simulink subsystem "PvtSubSys_AHBC"  (R2020b)
settings: Solver=VariableStepAuto  StartTime=0.0  StopTime=10.0  RelTol=1e-3
undefined symbols (not defined in the file): P_AHBC_ABS_ENABLE, P_AHBC_DRIVE_DIRECTION_ENABLE, P_AHBC_ESP_ENABLE, P_AHBC_FOG_ENABLE, P_AHBC_FOG_TIME, P_AHBC_HIGHBEAM_ACTIVE_GRACE, P_AHBC_LAT_ACC_ENTER, P_AHBC_LAT_ACC_EXIT, P_AHBC_MAX_ONCOMING_DISTANCE_COUPLE2, P_AHBC_MAX_ONCOMING_DISTANCE_ONE2, P_AHBC_MAX_TAILLIGHT_DISTANCE_COUPLE2, P_AHBC_MAX_TAILLIGHT_DISTANCE_ONE2, P_AHBC_SPEED_SWITCH_HIGH_BEAM_OFF2, P_AHBC_SPEED_SWITCH_HIGH_BEAM_ON2, P_AHBC_TrafficStyle, P_AHBC_TURN_LAMP_ENABLE, P_AHBC_WIPER_ENABLE, P_AHBC_WIPER_TIME, P_AHBC_YAW_RATE_ENTER, P_AHBC_YAW_RATE_EXIT
libraries: simulink x57
(part 3 of 4)

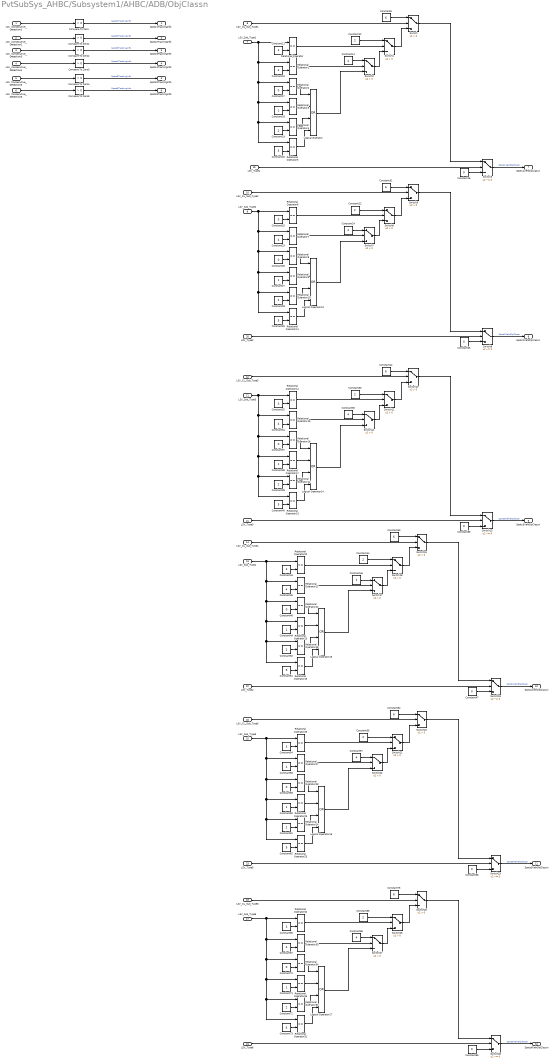
== system PvtSubSys_AHBC/Subsystem1/AHBC/ADB/ObjClassn ==
  LSV_Consecutive_Detection1 : Inport
  LSV_Consecutive_Detection2 : Inport  Port=2
  LSV_Consecutive_Detection3 : Inport  Port=3
  LSV_Consecutive_Detection4 : Inport  Port=4
  LSV_Consecutive_Detection5 : Inport  Port=5
  LSV_Consecutive_Detection6 : Inport  Port=6
  LSV_Sub_Type1 : Inport  Port=7
  LSV_CL_Sub_Type1 : Inport  Port=8
  LSV_Sub_Type2 : Inport  Port=9
  LSV_CL_Sub_Type2 : Inport  Port=10
  LSV_Sub_Type3 : Inport  Port=11
  LSV_CL_Sub_Type3 : Inport  Port=12
  LSV_Sub_Type4 : Inport  Port=13
  LSV_CL_Sub_Type4 : Inport  Port=14
  LSV_Sub_Type5 : Inport  Port=15
  LSV_CL_Sub_Type5 : Inport  Port=16
  LSV_Sub_Type6 : Inport  Port=17
  LSV_CL_Sub_Type6 : Inport  Port=18
  LSV_Type1 : Inport  Port=19
  LSV_Type2 : Inport  Port=20
  LSV_Type3 : Inport  Port=21
  LSV_Type4 : Inport  Port=22
  LSV_Type5 : Inport  Port=23
  LSV_Type6 : Inport  Port=24
  Compare To Zero{,1..5} (6 alike) : simulink/Logic and Bit Operations/Compare To Zero  relop=>  OutDataTypeStr=boolean
  Constant{11,15,32,43,54,65} (6 alike) : Constant  Value=3
  Constant{12,19,22,28,33,39,44,50,55,61,66,72} (12 alike) : Constant  Value=2
  Constant{13..14,23..24,34..35,45..46,56..57,67..68} (12 alike) : Constant  Value=4
  Constant{16..17,25..26,36..37,47..48,58..59,69..70} (12 alike) : Constant  Value=0
  Constant{18,27,38,49,60,71} (6 alike) : Constant
  Constant{20,29,40,51,62,73} (6 alike) : Constant  Value=5
  Constant{6,31,42,53,64,75} (6 alike) : Constant  Value=6
  Logical Operator{,13..17} (6 alike) : Logic  Operator=OR  Inputs=4  AllPortsSameDT=off  OutDataTypeStr=boolean
  Relational Operator{,1..35} (36 alike) : RelationalOperator  Operator===  OutDataTypeStr=boolean  RndMeth=Simplest
  Switch{,1..2,5..7,10..12,15..17,20..22,25..27} (18 alike) : Switch  Criteria=u2 > Threshold  OutDataTypeStr=uint8
  Switch{3,8,13,18,23,28} (6 alike) : Switch  Criteria=u2 ~= 0  OutDataTypeStr=uint8
  Spots1TrackingInfo : Outport  OutDataTypeStr=boolean  PortDimensions=1
  Spots2TrackingInfo : Outport  Port=2  OutDataTypeStr=boolean  PortDimensions=1
  Spots3TrackingInfo : Outport  Port=3  OutDataTypeStr=boolean  PortDimensions=1
  Spots4TrackingInfo : Outport  Port=4  OutDataTypeStr=boolean  PortDimensions=1
  Spots5TrackingInfo : Outport  Port=5  OutDataTypeStr=boolean  PortDimensions=1
  Spots6TrackingInfo : Outport  Port=6  OutDataTypeStr=boolean  PortDimensions=1
  Spots1VehObjClassn : Outport  Port=7  OutDataTypeStr=uint8  PortDimensions=1
  Spots2VehObjClassn : Outport  Port=8  OutDataTypeStr=uint8  PortDimensions=1
  Spots3VehObjClassn : Outport  Port=9  OutDataTypeStr=uint8  PortDimensions=1
  Spots4VehObjClassn : Outport  Port=10  OutDataTypeStr=uint8  PortDimensions=1
  Spots5VehObjClassn : Outport  Port=11  OutDataTypeStr=uint8  PortDimensions=1
  Spots6VehObjClassn : Outport  Port=12  OutDataTypeStr=uint8  PortDimensions=1
  wires:
  LSV_Consecutive_Detection4/1 -> Compare To Zero3/1
  Compare To Zero3/1 -> Spots4TrackingInfo/1  "Spots4TrackingInfo"
  Compare To Zero4/1 -> Spots5TrackingInfo/1  "Spots5TrackingInfo"
  LSV_Consecutive_Detection5/1 -> Compare To Zero4/1
  LSV_Consecutive_Detection6/1 -> Compare To Zero5/1
  Compare To Zero5/1 -> Spots6TrackingInfo/1  "Spots6TrackingInfo"
  Compare To Zero2/1 -> Spots3TrackingInfo/1  "Spots3TrackingInfo"
  LSV_Consecutive_Detection3/1 -> Compare To Zero2/1
  LSV_Consecutive_Detection2/1 -> Compare To Zero1/1
  Compare To Zero1/1 -> Spots2TrackingInfo/1  "Spots2TrackingInfo"
  Compare To Zero/1 -> Spots1TrackingInfo/1  "Spots1TrackingInfo"
  LSV_Consecutive_Detection1/1 -> Compare To Zero/1
  Logical Operator17/1 -> Switch27/3
  Logical Operator16/1 -> Switch22/3
  Logical Operator15/1 -> Switch17/3
  Logical Operator14/1 -> Switch12/3
  Logical Operator13/1 -> Switch7/3
  Logical Operator/1 -> Switch2/3
  Constant69/1 -> Switch28/3
  Switch21/1 -> Switch20/3
  Relational Operator29/1 -> Logical Operator16/2
  Relational Operator28/1 -> Logical Operator16/1
  Switch28/1 -> Spots6VehObjClassn/1  "Spots6VehObjClassn"
  Constant31/1 -> Switch5/1
  Relational Operator34/1 -> Logical Operator17/1
  LSV_Type4/1 -> Switch18/2
  Relational Operator30/1 -> Logical Operator17/3
  Constant71/1 -> Relational Operator35/2
  Constant56/1 -> Relational Operator27/2
  Relational Operator24/1 -> Logical Operator16/3
  Constant61/1 -> Relational Operator24/2
  Relational Operator22/1 -> Logical Operator15/1
  Switch22/1 -> Switch21/3
  Constant73/1 -> Relational Operator31/2
  Switch6/1 -> Switch5/3
  Relational Operator9/1 -> Logical Operator13/2
  Constant54/1 -> Relational Operator26/2
  Constant64/1 -> Switch20/1
  Constant24/1 -> Switch7/1
  Constant53/1 -> Switch15/1
  Switch15/1 -> Switch18/1
  Constant45/1 -> Relational Operator21/2
  Switch23/1 -> Spots5VehObjClassn/1  "Spots5VehObjClassn"
  Switch16/1 -> Switch15/3
  Constant47/1 -> Switch18/3
  Constant48/1 -> Relational Operator22/2
  Relational Operator13/1 -> Logical Operator14/4
  LSV_CL_Sub_Type5/1 -> Switch20/2
  Relational Operator12/1 -> Logical Operator14/3
  Relational Operator16/1 -> Logical Operator14/1
  Relational Operator17/1 -> Logical Operator14/2
  Relational Operator4/1 -> Logical Operator/3
  Constant58/1 -> Switch23/3
  Relational Operator18/1 -> Logical Operator15/3
  Constant36/1 -> Switch13/3
  LSV_CL_Sub_Type6/1 -> Switch25/2
  LSV_Type6/1 -> Switch28/2
  Relational Operator23/1 -> Logical Operator15/2
  Constant38/1 -> Relational Operator17/2
  Constant65/1 -> Relational Operator32/2
  Constant70/1 -> Relational Operator34/2
  LSV_Sub_Type2/1 -> Relational Operator6/1, Relational Operator7/1, Relational Operator8/1, Relational Operator9/1, Relational Operator11/1, Relational Operator10/1
  LSV_Type1/1 -> Switch3/2
  Constant62/1 -> Relational Operator25/2
  LSV_Sub_Type6/1 -> Relational Operator32/1, Relational Operator33/1, Relational Operator34/1, Relational Operator35/1, Relational Operator31/1, Relational Operator30/1
  Constant23/1 -> Relational Operator7/2
  Relational Operator27/1 -> Switch22/2
  Constant26/1 -> Relational Operator8/2
  LSV_Type3/1 -> Switch13/2
  Constant6/1 -> Switch/1
  Relational Operator31/1 -> Logical Operator17/4
  Constant50/1 -> Relational Operator18/2
  LSV_CL_Sub_Type2/1 -> Switch5/2
  Constant20/1 -> Relational Operator5/2
  Constant68/1 -> Switch27/1
  LSV_Type5/1 -> Switch23/2
  Relational Operator10/1 -> Logical Operator13/3
  Constant32/1 -> Relational Operator14/2
  Relational Operator21/1 -> Switch17/2
  Switch11/1 -> Switch10/3
  Constant46/1 -> Switch17/1
  Switch27/1 -> Switch26/3
  Constant60/1 -> Relational Operator29/2
  Constant72/1 -> Relational Operator30/2
  Relational Operator8/1 -> Logical Operator13/1
  Constant57/1 -> Switch22/1
  Constant25/1 -> Switch8/3
  Constant16/1 -> Switch3/3
  Switch7/1 -> Switch6/3
  Switch5/1 -> Switch8/1
  Switch18/1 -> Spots4VehObjClassn/1  "Spots4VehObjClassn"
  Switch20/1 -> Switch23/1
  Constant39/1 -> Relational Operator12/2
  Constant33/1 -> Switch11/1
  Constant37/1 -> Relational Operator16/2
  LSV_Sub_Type1/1 -> Relational Operator4/1, Relational Operator5/1, Relational Operator3/1, Relational Operator2/1, Relational Operator1/1, Relational Operator/1
  Constant42/1 -> Switch10/1
  Relational Operator25/1 -> Logical Operator16/4
  Switch13/1 -> Spots3VehObjClassn/1  "Spots3VehObjClassn"
  Constant27/1 -> Relational Operator9/2
  Relational Operator15/1 -> Switch12/2
  Switch17/1 -> Switch16/3
  Constant22/1 -> Switch6/1
  LSV_Sub_Type4/1 -> Relational Operator20/1, Relational Operator21/1, Relational Operator22/1, Relational Operator23/1, Relational Operator19/1, Relational Operator18/1
  Constant15/1 -> Relational Operator6/2
  Switch26/1 -> Switch25/3
  Relational Operator7/1 -> Switch7/2
  Constant28/1 -> Relational Operator10/2
  Constant67/1 -> Relational Operator33/2
  Constant44/1 -> Switch16/1
  Relational Operator11/1 -> Logical Operator13/4
  Constant51/1 -> Relational Operator19/2
  Constant12/1 -> Switch1/1
  Relational Operator5/1 -> Logical Operator/4
  Relational Operator3/1 -> Logical Operator/2
  Constant43/1 -> Relational Operator20/2
  LSV_Type2/1 -> Switch8/2
  Switch10/1 -> Switch13/1
  Constant19/1 -> Relational Operator4/2
  Relational Operator33/1 -> Switch27/2
  Switch3/1 -> Spots1VehObjClassn/1  "Spots1VehObjClassn"
  Relational Operator6/1 -> Switch6/2
  Constant35/1 -> Switch12/1
  Switch12/1 -> Switch11/3
  Relational Operator2/1 -> Logical Operator/1
  Switch8/1 -> Spots2VehObjClassn/1  "Spots2VehObjClassn"
  Relational Operator32/1 -> Switch26/2
  Relational Operator26/1 -> Switch21/2
  Constant18/1 -> Relational Operator3/2
  Relational Operator19/1 -> Logical Operator15/4
  Relational Operator14/1 -> Switch11/2
  Switch1/1 -> Switch/3
  Constant17/1 -> Relational Operator2/2
  Constant40/1 -> Relational Operator13/2
  LSV_Sub_Type3/1 -> Relational Operator12/1, Relational Operator13/1, Relational Operator17/1, Relational Operator16/1, Relational Operator15/1, Relational Operator14/1
  Constant49/1 -> Relational Operator23/2
  Constant14/1 -> Switch2/1
  Switch2/1 -> Switch1/3
  Relational Operator20/1 -> Switch16/2
  LSV_CL_Sub_Type3/1 -> Switch10/2
  Constant55/1 -> Switch21/1
  Constant75/1 -> Switch25/1
  Constant66/1 -> Switch26/1
  Switch/1 -> Switch3/1
  Constant11/1 -> Relational Operator/2
  LSV_CL_Sub_Type1/1 -> Switch/2
  LSV_CL_Sub_Type4/1 -> Switch15/2
  Relational Operator35/1 -> Logical Operator17/2
  Constant13/1 -> Relational Operator1/2
  Constant59/1 -> Relational Operator28/2
  Constant34/1 -> Relational Operator15/2
  Switch25/1 -> Switch28/1
  Relational Operator/1 -> Switch1/2
  Constant29/1 -> Relational Operator11/2
  LSV_Sub_Type5/1 -> Relational Operator24/1, Relational Operator25/1, Relational Operator29/1, Relational Operator28/1, Relational Operator27/1, Relational Operator26/1
  Relational Operator1/1 -> Switch2/2

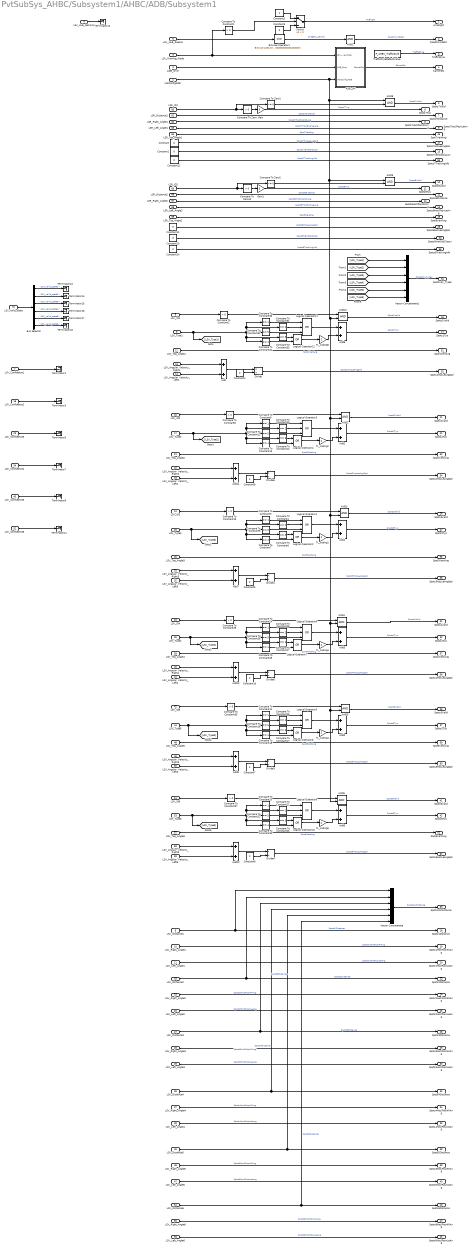
== system PvtSubSys_AHBC/Subsystem1/AHBC/ADB/Subsystem1 ==
  VehConfigADB : Inport
  ADB_error : Inport  Port=2
  LSV_Running_Mode : Inport  Port=3
  LSV_HLB_Decision : Inport  Port=4
  LSV_HLB_Reason : Inport  Port=5
  LSV_ID1 : Inport  Port=6
  LSV_Confidence1 : Inport  Port=7
  LSV_Type1 : Inport  Port=8
  LSV_Distance1 : Inport  Port=9  OutDataTypeStr=uint16
  LSV_Right_Angle1 : Inport  Port=10
  LSV_Left_Angle1 : Inport  Port=11
  LSV_Top_Angle1 : Inport  Port=12
  LSV_Angular_Velocity_Right1 : Inport  Port=13
  LSV_Angular_Velocity_Left1 : Inport  Port=14
  LSV_ID2 : Inport  Port=15
  LSV_Confidence2 : Inport  Port=16
  LSV_Type2 : Inport  Port=17
  LSV_Distance2 : Inport  Port=18  OutDataTypeStr=uint16
  LSV_Right_Angle2 : Inport  Port=19
  LSV_Left_Angle2 : Inport  Port=20
  LSV_Top_Angle2 : Inport  Port=21
  LSV_Angular_Velocity_Right2 : Inport  Port=22
  LSV_Angular_Velocity_Left2 : Inport  Port=23
  LSV_ID3 : Inport  Port=24
  LSV_Confidence3 : Inport  Port=25
  LSV_Type3 : Inport  Port=26
  LSV_Distance3 : Inport  Port=27  OutDataTypeStr=uint16
  LSV_Right_Angle3 : Inport  Port=28
  LSV_Left_Angle3 : Inport  Port=29
  LSV_Top_Angle3 : Inport  Port=30
  LSV_Angular_Velocity_Right3 : Inport  Port=31
  LSV_Angular_Velocity_Left3 : Inport  Port=32
  LSV_ID4 : Inport  Port=33
  LSV_Confidence4 : Inport  Port=34
  LSV_Type4 : Inport  Port=35
  LSV_Distance4 : Inport  Port=36  OutDataTypeStr=uint16
  LSV_Right_Angle4 : Inport  Port=37
  LSV_Left_Angle4 : Inport  Port=38
  LSV_Top_Angle4 : Inport  Port=39
  LSV_Angular_Velocity_Right4 : Inport  Port=40
  LSV_Angular_Velocity_Left4 : Inport  Port=41
  LSV_ID5 : Inport  Port=42
  LSV_Confidence5 : Inport  Port=43
  LSV_Type5 : Inport  Port=44
  LSV_Distance5 : Inport  Port=45  OutDataTypeStr=uint16
  LSV_Right_Angle5 : Inport  Port=46
  LSV_Left_Angle5 : Inport  Port=47
  LSV_Top_Angle5 : Inport  Port=48
  LSV_Angular_Velocity_Right5 : Inport  Port=49
  LSV_Angular_Velocity_Left5 : Inport  Port=50
  LSV_ID6 : Inport  Port=51
  LSV_Confidence6 : Inport  Port=52
  LSV_Type6 : Inport  Port=53
  LSV_Distance6 : Inport  Port=54  OutDataTypeStr=uint16
  LSV_Right_Angle6 : Inport  Port=55
  LSV_Left_Angle6 : Inport  Port=56
  LSV_Top_Angle6 : Inport  Port=57
  LSV_Angular_Velocity_Right6 : Inport  Port=58
  LSV_Angular_Velocity_Left6 : Inport  Port=59
  LSR_ID1 : Inport  Port=60
  LSR_Distance1 : Inport  Port=61  OutDataTypeStr=uint16
  LSR_Right_Angle1 : Inport  Port=62
  LSR_Left_Angle1 : Inport  Port=63
  LSR_Top_Angle1 : Inport  Port=64
  LSR_ID2 : Inport  Port=65
  LSR_Distance2 : Inport  Port=66  OutDataTypeStr=uint16
  LSR_Right_Angle2 : Inport  Port=67
  LSR_Left_Angle2 : Inport  Port=68
  LSR_Top_Angle2 : Inport  Port=69
  LSV_valid_state : Inport  Port=70
  ADB_SM : Stateflow chart  TreatAsAtomicUnit=on
  AND1 : Logic  Inputs=1  AllPortsSameDT=off  OutDataTypeStr=boolean
  AND{2..6,8..10} (8 alike) : Logic  AllPortsSameDT=off  OutDataTypeStr=boolean
  Add{,1..7,9..12} (12 alike) : Sum
  Bitwise Operator1 : simulink/Logic and Bit Operations/Bitwise Operator  logicop=AND  UseBitMask=on  BitMask=bin2dec('00000000000000000000000000100000')  BitMaskRealWorld=Stored Integer
  Bus Selector : BusSelector  OutputSignals=LSV_valid_state1,LSV_valid_state2,LSV_valid_state3,LSV_valid_state4,LSV_valid_state5,LSV_valid_state6
  Compare To Constant{1..2,8,19,29,35,37} (7 alike) : simulink/Logic and Bit Operations/Compare To Constant  relop=>  const=0  OutDataTypeStr=boolean
  Compare To Constant{4,10,15,21,25,31} (6 alike) : simulink/Logic and Bit Operations/Compare To Constant  relop===  const=2  OutDataTypeStr=boolean
  Compare To Constant{5,11,16,22,26,32} (6 alike) : simulink/Logic and Bit Operations/Compare To Constant  relop===  const=5  OutDataTypeStr=boolean
  Compare To Constant{6,12,17,23,27,33} (6 alike) : simulink/Logic and Bit Operations/Compare To Constant  relop===  const=3  OutDataTypeStr=boolean
  Compare To Constant{7,13,18,28,30,34} (6 alike) : simulink/Logic and Bit Operations/Compare To Constant  relop===  const=4  OutDataTypeStr=boolean
  Compare To Constant{3,9,14,20,24,36} (6 alike) : simulink/Logic and Bit Operations/Compare To Constant  relop===  const=1  OutDataTypeStr=boolean
  Compare To Zero : simulink/Logic and Bit Operations/Compare To Zero  relop=>  OutDataTypeStr=boolean
  Compare To Zero1 : simulink/Logic and Bit Operations/Compare To Zero  relop=~=  OutDataTypeStr=boolean
  Compare To Zero10 : simulink/Logic and Bit Operations/Compare To Zero  relop=>  OutDataTypeStr=boolean
  Compare To Zero2 : simulink/Logic and Bit Operations/Compare To Zero  relop=~=  OutDataTypeStr=boolean
  Constant : Constant  Value=0  OutDataTypeStr=single
  Constant1 : Constant  Value=0  OutDataTypeStr=uint8
  Constant{4..5,7..10} (6 alike) : Constant  Value=2  OutDataTypeStr=single
  Constant11 : Constant  Value=0  OutDataTypeStr=boolean
  Constant12 : Constant  Value=0  OutDataTypeStr=single
  Constant13 : Constant  Value=0  OutDataTypeStr=uint8
  Constant14 : Constant  Value=0  OutDataTypeStr=boolean
  Constant2 : Constant  OutDataTypeStr=boolean
  Constant3 : Constant  Value=0  OutDataTypeStr=boolean
  Divide{,1,3..6} (6 alike) : Product  Inputs=*/  OutDataTypeStr=single
  Gain : Gain  Gain=3  OutDataTypeStr=uint8
  Gain1 : Gain  Gain=3  OutDataTypeStr=uint8
  Logical Operator{1,3,5..6,9,11} (6 alike) : Logic  Operator=OR  Inputs=3  AllPortsSameDT=off  OutDataTypeStr=boolean
  Logical Operator{2,4,7..8,10,12} (6 alike) : Logic  Operator=OR  AllPortsSameDT=off  OutDataTypeStr=boolean
  Switch : Switch  Criteria=u2 > Threshold
  TL_coding{1..6} (6 alike) : Gain  Gain=2  OutDataTypeStr=uint8
  Terminator{1,3,5,7,9,11..18} (13 alike) : Terminator
  TrafficStyleDefaultValue : Constant  Value=P_AHBC_TrafficStyle  OutDataTypeStr=uint8
  Vector Concatenate : Concatenate  NumInputs=6
  Vector Concatenate1 : Concatenate  NumInputs=6
  AmBlight : Outport  OutDataTypeStr=boolean  PortDimensions=1
  RoadIllumDetd : Outport  Port=2  PortDimensions=1
  TrafficStyle : Outport  Port=3  OutDataTypeStr=uint8  PortDimensions=1
  CamerSts : Outport  Port=4  PortDimensions=1
  Spots7Valid : Outport  Port=5  PortDimensions=1
  Spots7Typ : Outport  Port=6  PortDimensions=1
  Spots7Distance : Outport  Port=7  PortDimensions=1
  Spots7HozlPosnRiAng : Outport  Port=8  PortDimensions=1
  Spots7HozlPosnLeAng : Outport  Port=9  PortDimensions=1
  Spots8Valid : Outport  Port=10  PortDimensions=1
  Spots8Typ : Outport  Port=11  PortDimensions=1
  Spots8Distance : Outport  Port=12  PortDimensions=1
  Spots7VehObjClassn : Outport  Port=13  PortDimensions=1
  Spots8HozlPosnRiAng : Outport  Port=14  PortDimensions=1
  Spots8HozlPosnLeAng : Outport  Port=15  PortDimensions=1
  Spots1Valid : Outport  Port=16  PortDimensions=1
  Spots1Typ : Outport  Port=17  PortDimensions=1
  Spots1Distance : Outport  Port=18  PortDimensions=1
  Spots1HozlPosnRiAng : Outport  Port=19  PortDimensions=1
  Spots1HozlPosnLeAng : Outport  Port=20  OutDataTypeStr=single  PortDimensions=1
  Spots2Valid : Outport  Port=21  PortDimensions=1
  Spots2Typ : Outport  Port=22  PortDimensions=1
  Spots2Distance : Outport  Port=23  PortDimensions=1
  Spots2HozlPosnRiAng : Outport  Port=24  PortDimensions=1
  Spots2HozlPosnLeAng : Outport  Port=25  PortDimensions=1
  Spots3Valid : Outport  Port=26  PortDimensions=1
  Spots3Typ : Outport  Port=27  PortDimensions=1
  Spots3Distance : Outport  Port=28  PortDimensions=1
  Spots3HozlPosnRiAng : Outport  Port=29  PortDimensions=1
  Spots3HozlPosnLeAng : Outport  Port=30  PortDimensions=1
  Spots4Valid : Outport  Port=31  PortDimensions=1
  Spots4Typ : Outport  Port=32  PortDimensions=1
  Spots4Distance : Outport  Port=33  PortDimensions=1
  Spots4HozlPosnRiAng : Outport  Port=34  PortDimensions=1
  Spots4HozlPosnLeAng : Outport  Port=35  PortDimensions=1
  Spots5Valid : Outport  Port=36  PortDimensions=1
  Spots5Typ : Outport  Port=37  PortDimensions=1
  Spots5Distance : Outport  Port=38  PortDimensions=1
  Spots5HozlPosnRiAng : Outport  Port=39  PortDimensions=1
  Spots5HozlPosnLeAng : Outport  Port=40  PortDimensions=1
  Spots6Valid : Outport  Port=41  PortDimensions=1
  Spots6Typ : Outport  Port=42  PortDimensions=1
  Spots6Distance : Outport  Port=43  PortDimensions=1
  Spots6HozlPosnRiAng : Outport  Port=44  PortDimensions=1
  Spots6HozlPosnLeAng : Outport  Port=45  PortDimensions=1
  Spot7VertAng : Outport  Port=46  PortDimensions=1
  Spots7HozLeAngSpd : Outport  Port=47  PortDimensions=1
  Spots8HozLeAngSpd : Outport  Port=48  PortDimensions=1
  Spot8VertAng : Outport  Port=49  PortDimensions=1
  Spots8VehObjClassn : Outport  Port=50  PortDimensions=1
  Spot1VertAng : Outport  Port=51  PortDimensions=1
  Spots1HozLeAngSpd : Outport  Port=52  OutDataTypeStr=single  PortDimensions=1
  Spot2VertAng : Outport  Port=53  PortDimensions=1
  Spots2HozLeAngSpd : Outport  Port=54  OutDataTypeStr=single  PortDimensions=1
  Spot3VertAng : Outport  Port=55  PortDimensions=1
  Spots3HozLeAngSpd : Outport  Port=56  OutDataTypeStr=single  PortDimensions=1
  Spot4VertAng : Outport  Port=57  PortDimensions=1
  Spots4HozLeAngSpd : Outport  Port=58  OutDataTypeStr=single  PortDimensions=1
  Spot5VertAng : Outport  Port=59  PortDimensions=1
  Spots5HozLeAngSpd : Outport  Port=60  OutDataTypeStr=single  PortDimensions=1
  Spot6VertAng : Outport  Port=61  PortDimensions=1
  Spots6HozLeAngSpd : Outport  Port=62  OutDataTypeStr=single  PortDimensions=1
  SpotsLSVDistance : Outport  Port=63  PortDimensions=6
  SpotsLSV_Types : Outport  Port=64  PortDimensions=6
  Spots7TrackingInfo : Outport  Port=65  OutDataTypeStr=boolean  PortDimensions=1
  Spots8TrackingInfo : Outport  Port=66  OutDataTypeStr=boolean  PortDimensions=1
  wires:
  Compare To Constant37/1 -> AND6/1
  Compare To Constant35/1 -> AND5/1
  Compare To Constant29/1 -> AND4/1
  Compare To Constant19/1 -> AND3/1
  Compare To Constant8/1 -> AND2/1
  LSV_HLB_Decision/1 -> Terminator12/1
  LSV_Confidence6/1 -> Terminator11/1
  LSV_Confidence5/1 -> Terminator9/1
  LSV_Confidence4/1 -> Terminator7/1
  LSV_Confidence3/1 -> Terminator5/1
  LSV_Confidence2/1 -> Terminator3/1
  LSV_Confidence1/1 -> Terminator1/1
  LSV_ID1/1 -> Compare To Constant2/1
  LSV_ID6/1 -> Compare To Constant37/1
  LSV_ID2/1 -> Compare To Constant8/1
  LSV_ID5/1 -> Compare To Constant35/1
  LSV_ID4/1 -> Compare To Constant29/1
  LSV_ID3/1 -> Compare To Constant19/1
  Compare To Constant2/1 -> AND10/1
  Bus Selector/6 -> Terminator18/1  "<LSV_valid_state6>"
  Bus Selector/5 -> Terminator17/1  "<LSV_valid_state5>"
  Bus Selector/4 -> Terminator16/1  "<LSV_valid_state4>"
  Bus Selector/3 -> Terminator15/1  "<LSV_valid_state3>"
  Bus Selector/2 -> Terminator14/1  "<LSV_valid_state2>"
  Bus Selector/1 -> Terminator13/1  "<LSV_valid_state1>"
  LSV_valid_state/1 -> Bus Selector/1
  Constant11/1 -> Spots7TrackingInfo/1  "Spots7TrackingInfo"
  Constant14/1 -> Spots8TrackingInfo/1  "Spots8TrackingInfo"
  AND2/1 -> Spots2Valid/1  "Spots2Valid"
  Compare To Constant25/1 -> Logical Operator6/2
  Logical Operator2/1 -> TL_coding1/1
  Compare To Constant24/1 -> Logical Operator6/1
  TL_coding6/1 -> Add6/2
  Logical Operator6/1 -> Add3/1
  LSV_Left_Angle6/1 -> Spots6HozlPosnLeAng/1  "Spots6HozlPosnLeAng"
  Compare To Zero/1 -> Gain/1
  TL_coding2/1 -> Add2/2
  Compare To Zero10/1 -> Gain1/1
  Add/1 -> Divide/1
  Constant4/1 -> Divide/2
  Divide/1 -> Spots1HozLeAngSpd/1  "Spots1HozLeAngSpd"
  LSV_Angular_Velocity_Right1/1 -> Add/1
  LSV_Distance4/1 -> Vector Concatenate/4, Spots4Distance/1  "Spots4Distance"
  LSV_Top_Angle1/1 -> Spot1VertAng/1  "Spot1VertAng"
  LSV_Type5/1 -> Compare To Constant15/1, Compare To Constant14/1, Compare To Constant17/1, Compare To Constant18/1, Compare To Constant16/1, [LSV_Type5]
  LSR_Top_Angle1/1 -> Spot7VertAng/1  "Spot7VertAng"
  Vector Concatenate/1 -> SpotsLSVDistance/1  "SpotsLSVDistance"
  Compare To Constant30/1 -> Logical Operator10/2
  Compare To Zero2/1 -> AND9/2
  Compare To Constant13/1 -> Logical Operator4/2
  Add4/1 -> Spots5Typ/1  "Spots5Typ"
  TrafficStyleDefaultValue/1 -> TrafficStyle/1  "TrafficStyle"
  AND1/1 -> RoadIllumDetd/1  "RoadIllumDetd"
  Compare To Constant26/1 -> Logical Operator6/3
  AND5/1 -> Spots5Valid/1  "Spots5Valid"
  LSV_Distance2/1 -> Vector Concatenate/2, Spots2Distance/1  "Spots2Distance"
  AND4/1 -> Spots4Valid/1  "Spots4Valid"
  LSV_Right_Angle6/1 -> Spots6HozlPosnRiAng/1  "Spots6HozlPosnRiAng"
  LSV_Left_Angle4/1 -> Spots4HozlPosnLeAng/1  "Spots4HozlPosnLeAng"
  LSV_Running_Mode/1 -> ADB_SM/1(LSV_Running_Mode), Compare To Constant1/1
  LSV_Distance3/1 -> Vector Concatenate/3, Spots3Distance/1  "Spots3Distance"
  Compare To Constant36/1 -> Logical Operator11/1
  LSV_Right_Angle4/1 -> Spots4HozlPosnRiAng/1  "Spots4HozlPosnRiAng"
  Add2/1 -> Spots2Typ/1  "Spots2Typ"
  LSV_Right_Angle5/1 -> Spots5HozlPosnRiAng/1  "Spots5HozlPosnRiAng"
  Logical Operator12/1 -> TL_coding6/1
  Gain1/1 -> Spots8Typ/1  "Spots8Typ"
  Add3/1 -> Spots4Typ/1  "Spots4Typ"
  Compare To Constant33/1 -> Logical Operator12/1
  Vector Concatenate1/1 -> SpotsLSV_Types/1  "SpotsLSV_Types"
  Compare To Constant22/1 -> Logical Operator9/3
  Compare To Constant15/1 -> Logical Operator5/2
  Logical Operator1/1 -> Add1/1
  Compare To Constant34/1 -> Logical Operator12/2
  Constant9/1 -> Divide5/2
  Compare To Constant20/1 -> Logical Operator9/1
  Divide5/1 -> Spots2HozLeAngSpd/1  "Spots2HozLeAngSpd"
  Compare To Constant7/1 -> Logical Operator2/2
  Compare To Constant31/1 -> Logical Operator11/2
  Compare To Constant4/1 -> Logical Operator1/2
  Logical Operator7/1 -> TL_coding3/1
  Compare To Constant12/1 -> Logical Operator4/1
  Compare To Constant27/1 -> Logical Operator7/1
  Compare To Constant21/1 -> Logical Operator9/2
  LSV_Top_Angle4/1 -> Spot4VertAng/1  "Spot4VertAng"
  Compare To Constant10/1 -> Logical Operator3/2
  LSV_Right_Angle3/1 -> Spots3HozlPosnRiAng/1  "Spots3HozlPosnRiAng"
  Logical Operator8/1 -> TL_coding4/1
  LSV_Angular_Velocity_Left2/1 -> Add11/2
  LSV_Left_Angle5/1 -> Spots5HozlPosnLeAng/1  "Spots5HozlPosnLeAng"
  LSV_Left_Angle2/1 -> Spots2HozlPosnLeAng/1  "Spots2HozlPosnLeAng"
  [LSV_Type6] -> Vector Concatenate1/6
  Logical Operator9/1 -> Add5/1
  LSV_Top_Angle2/1 -> Spot2VertAng/1  "Spot2VertAng"
  Compare To Constant5/1 -> Logical Operator1/3
  Add5/1 -> Spots6Typ/1  "Spots6Typ"
  LSV_Type6/1 -> Compare To Constant22/1, Compare To Constant30/1, Compare To Constant23/1, Compare To Constant20/1, Compare To Constant21/1, [LSV_Type6]
  LSV_Top_Angle5/1 -> Spot5VertAng/1  "Spot5VertAng"
  AND8/1 -> Spots7Valid/1  "Spots7Valid"
  Compare To Constant28/1 -> Logical Operator7/2
  LSV_Type3/1 -> Compare To Constant4/1, Compare To Constant3/1, Compare To Constant6/1, Compare To Constant7/1, Compare To Constant5/1, [LSV_Type3]
  Bitwise Operator1/1 -> AND1/1  "STREET_LIGHTS"
  Compare To Constant11/1 -> Logical Operator3/3
  LSR_Right_Angle2/1 -> Spots8HozlPosnRiAng/1  "Spots8HozlPosnRiAng"
  LSV_Angular_Velocity_Right5/1 -> Add9/1
  Compare To Constant18/1 -> Logical Operator8/2
  TL_coding4/1 -> Add4/2
  LSV_Top_Angle3/1 -> Spot3VertAng/1  "Spot3VertAng"
  Compare To Zero1/1 -> AND8/2
  LSR_ID1/1 -> Compare To Zero1/1, Compare To Zero/1
  LSV_Left_Angle3/1 -> Spots3HozlPosnLeAng/1  "Spots3HozlPosnLeAng"
  Compare To Constant16/1 -> Logical Operator5/3
  Compare To Constant17/1 -> Logical Operator8/1
  LSV_Left_Angle1/1 -> Spots1HozlPosnLeAng/1  "Spots1HozlPosnLeAng"
  Compare To Constant14/1 -> Logical Operator5/1
  LSV_Angular_Velocity_Left6/1 -> Add10/2
  ADB_error/1 -> ADB_SM/2(ADB_Error)
  LSV_Angular_Velocity_Right6/1 -> Add10/1
  Constant1/1 -> Spots7VehObjClassn/1  "Spots7VehObjClassn"
  Constant7/1 -> Divide3/2
  Add11/1 -> Divide5/1
  Constant12/1 -> Spots8HozLeAngSpd/1  "Spots8HozLeAngSpd"
  AND3/1 -> Spots3Valid/1  "Spots3Valid"
  Divide1/1 -> Spots3HozLeAngSpd/1  "Spots3HozLeAngSpd"
  LSV_Distance1/1 -> Vector Concatenate/1, Spots1Distance/1  "Spots1Distance"
  Constant8/1 -> Divide4/2
  LSV_Right_Angle2/1 -> Spots2HozlPosnRiAng/1  "Spots2HozlPosnRiAng"
  [LSV_Type3] -> Vector Concatenate1/3
  Logical Operator4/1 -> TL_coding2/1
  [LSV_Type2] -> Vector Concatenate1/2
  LSV_Angular_Velocity_Left5/1 -> Add9/2
  Logical Operator3/1 -> Add2/1
  [LSV_Type5] -> Vector Concatenate1/5
  [LSV_Type4] -> Vector Concatenate1/4
  TL_coding3/1 -> Add3/2
  AND9/1 -> Spots8Valid/1  "Spots8Valid"
  LSV_Angular_Velocity_Left4/1 -> Add12/2
  Compare To Constant32/1 -> Logical Operator11/3
  Divide3/1 -> Spots5HozLeAngSpd/1  "Spots5HozLeAngSpd"
  Switch/1 -> AmBlight/1  "AmBlight"
  TL_coding1/1 -> Add1/2
  Compare To Constant23/1 -> Logical Operator10/1
  LSV_Type1/1 -> Compare To Constant32/1, Compare To Constant31/1, Compare To Constant36/1, Compare To Constant33/1, Compare To Constant34/1, [LSV_Type1]
  LSV_Angular_Velocity_Right3/1 -> Add7/1
  [LSV_Type1] -> Vector Concatenate1/1
  AND6/1 -> Spots6Valid/1  "Spots6Valid"
  Compare To Constant9/1 -> Logical Operator3/1
  Gain/1 -> Spots7Typ/1  "Spots7Typ"
  LSV_Angular_Velocity_Right2/1 -> Add11/1
  LSR_Top_Angle2/1 -> Spot8VertAng/1  "Spot8VertAng"
  Add6/1 -> Spots1Typ/1  "Spots1Typ"
  LSV_HLB_Reason/1 -> Bitwise Operator1/1
  Constant10/1 -> Divide6/2
  Constant/1 -> Spots7HozLeAngSpd/1  "Spots7HozLeAngSpd"
  LSR_ID2/1 -> Compare To Zero2/1, Compare To Zero10/1
  LSV_Distance5/1 -> Vector Concatenate/5, Spots5Distance/1  "Spots5Distance"
  Compare To Constant3/1 -> Logical Operator1/1
  LSR_Left_Angle2/1 -> Spots8HozlPosnLeAng/1  "Spots8HozlPosnLeAng"
  Divide6/1 -> Spots4HozLeAngSpd/1  "Spots4HozLeAngSpd"
  LSV_Type4/1 -> Compare To Constant26/1, Compare To Constant28/1, Compare To Constant27/1, Compare To Constant24/1, Compare To Constant25/1, [LSV_Type4]
  Add9/1 -> Divide3/1
  Logical Operator10/1 -> TL_coding5/1
  ADB_SM/1(CamerSts) -> CamerSts/1  "CamerSts"
  Constant13/1 -> Spots8VehObjClassn/1  "Spots8VehObjClassn"
  Constant5/1 -> Divide1/2
  Add12/1 -> Divide6/1
  LSV_Angular_Velocity_Left1/1 -> Add/2
  Compare To Constant6/1 -> Logical Operator2/1
  Add10/1 -> Divide4/1
  VehConfigADB/1 -> ADB_SM/3(VehConfigADB), AND9/1, AND2/2, AND3/2, AND5/2, AND6/2, AND4/2, AND10/2, AND8/1
  LSV_Angular_Velocity_Right4/1 -> Add12/1
  LSV_Right_Angle1/1 -> Spots1HozlPosnRiAng/1  "Spots1HozlPosnRiAng"
  Add1/1 -> Spots3Typ/1  "Spots3Typ"
  AND10/1 -> Spots1Valid/1  "Spots1Valid"
  LSR_Left_Angle1/1 -> Spots7HozlPosnLeAng/1  "Spots7HozlPosnLeAng"
  LSR_Distance2/1 -> Spots8Distance/1  "Spots8Distance"
  Divide4/1 -> Spots6HozLeAngSpd/1  "Spots6HozLeAngSpd"
  LSR_Distance1/1 -> Spots7Distance/1  "Spots7Distance"
  LSV_Distance6/1 -> Vector Concatenate/6, Spots6Distance/1  "Spots6Distance"
  Logical Operator5/1 -> Add4/1
  LSV_Type2/1 -> Compare To Constant13/1, Compare To Constant12/1, Compare To Constant11/1, Compare To Constant9/1, Compare To Constant10/1, [LSV_Type2]
  Logical Operator11/1 -> Add6/1
  Add7/1 -> Divide1/1
  LSV_Angular_Velocity_Left3/1 -> Add7/2
  LSV_Top_Angle6/1 -> Spot6VertAng/1  "Spot6VertAng"
  TL_coding5/1 -> Add5/2
  LSR_Right_Angle1/1 -> Spots7HozlPosnRiAng/1  "Spots7HozlPosnRiAng"
  Compare To Constant1/1 -> Switch/2
  Constant2/1 -> Switch/1
  Constant3/1 -> Switch/3

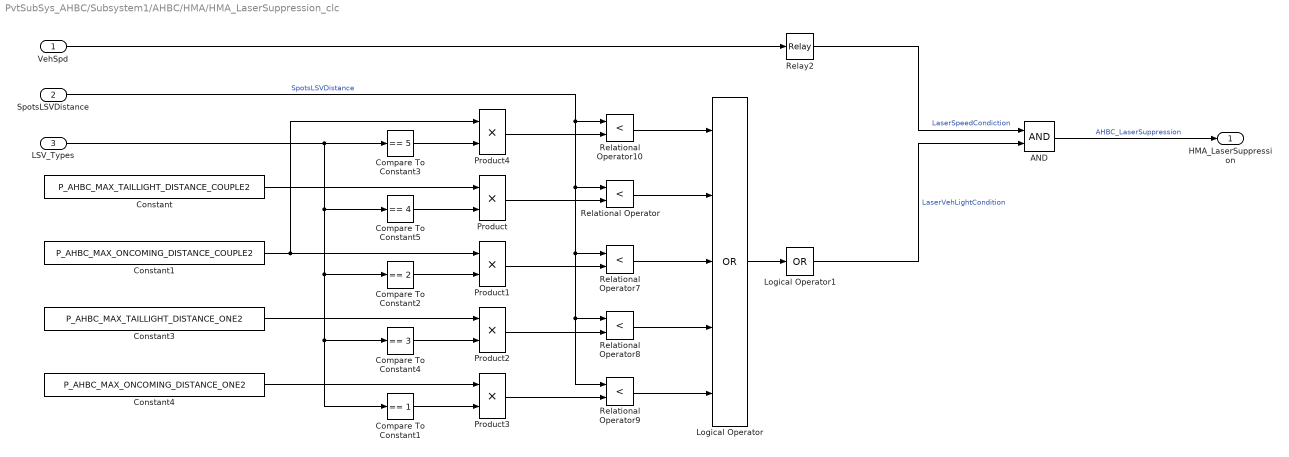
== system PvtSubSys_AHBC/Subsystem1/AHBC/HMA/HMA_LaserSuppression_clc ==
  VehSpd : Inport
  SpotsLSVDistance : Inport  Port=2
  LSV_Types : Inport  Port=3
  AND : Logic  AllPortsSameDT=off  OutDataTypeStr=boolean
  Compare To Constant1 : simulink/Logic and Bit Operations/Compare To Constant  relop===  const=1  OutDataTypeStr=boolean
  Compare To Constant2 : simulink/Logic and Bit Operations/Compare To Constant  relop===  const=2  OutDataTypeStr=boolean
  Compare To Constant3 : simulink/Logic and Bit Operations/Compare To Constant  relop===  const=5  OutDataTypeStr=boolean
  Compare To Constant4 : simulink/Logic and Bit Operations/Compare To Constant  relop===  const=3  OutDataTypeStr=boolean
  Compare To Constant5 : simulink/Logic and Bit Operations/Compare To Constant  relop===  const=4  OutDataTypeStr=boolean
  Constant : Constant  Value=P_AHBC_MAX_TAILLIGHT_DISTANCE_COUPLE2
  Constant1 : Constant  Value=P_AHBC_MAX_ONCOMING_DISTANCE_COUPLE2
  Constant3 : Constant  Value=P_AHBC_MAX_TAILLIGHT_DISTANCE_ONE2
  Constant4 : Constant  Value=P_AHBC_MAX_ONCOMING_DISTANCE_ONE2
  Logical Operator : Logic  Operator=OR  Inputs=5  AllPortsSameDT=off  OutDataTypeStr=boolean
  Logical Operator1 : Logic  Operator=OR  Inputs=1  AllPortsSameDT=off  OutDataTypeStr=boolean
  Product{,1..4} (5 alike) : Product
  Relational Operator{,7..10} (5 alike) : RelationalOperator  Operator=<  OutDataTypeStr=boolean  RndMeth=Simplest
  Relay2 : Relay  OnSwitchValue=P_AHBC_SPEED_SWITCH_HIGH_BEAM_ON2  OffSwitchValue=P_AHBC_SPEED_SWITCH_HIGH_BEAM_OFF2  OnOutputValue=true  OffOutputValue=false  OutDataTypeStr=boolean
  HMA_LaserSuppression : Outport
  wires:
  VehSpd/1 -> Relay2/1
  Relational Operator8/1 -> Logical Operator/4
  Product4/1 -> Relational Operator10/2
  Product3/1 -> Relational Operator9/2
  Product1/1 -> Relational Operator7/2
  Relational Operator7/1 -> Logical Operator/3
  AND/1 -> HMA_LaserSuppression/1  "AHBC_LaserSuppression"
  Constant1/1 -> Product4/1, Product1/1
  Compare To Constant2/1 -> Product1/2
  Logical Operator/1 -> Logical Operator1/1
  Constant3/1 -> Product2/1
  Logical Operator1/1 -> AND/2  "LaserVehLightCondition"
  Relay2/1 -> AND/1  "LaserSpeedCondiction"
  Relational Operator10/1 -> Logical Operator/1
  Relational Operator/1 -> Logical Operator/2
  Product2/1 -> Relational Operator8/2
  Compare To Constant1/1 -> Product3/2
  Product/1 -> Relational Operator/2
  Compare To Constant3/1 -> Product4/2
  Constant/1 -> Product/1
  Relational Operator9/1 -> Logical Operator/5
  SpotsLSVDistance/1 -> Relational Operator/1, Relational Operator7/1, Relational Operator8/1, Relational Operator9/1, Relational Operator10/1  "SpotsLSVDistance"
  Constant4/1 -> Product3/1
  LSV_Types/1 -> Compare To Constant3/1, Compare To Constant5/1, Compare To Constant2/1, Compare To Constant4/1, Compare To Constant1/1
  Compare To Constant5/1 -> Product/2
  Compare To Constant4/1 -> Product2/2

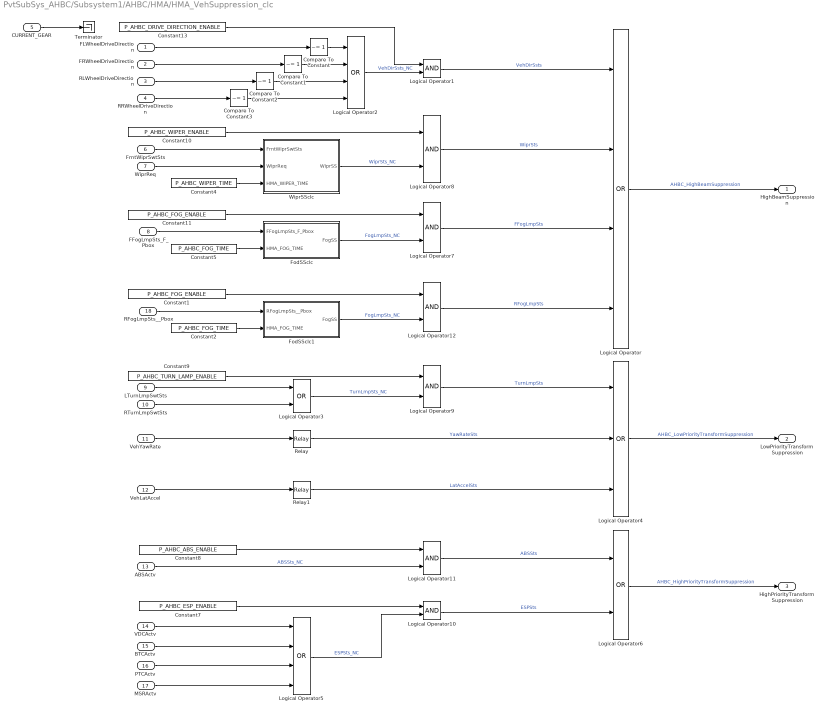
== system PvtSubSys_AHBC/Subsystem1/AHBC/HMA/HMA_VehSuppression_clc ==
  FLWheelDriveDirection : Inport
  FRWheelDriveDirection : Inport  Port=2
  RLWheelDriveDirection : Inport  Port=3
  RRWheelDriveDirection : Inport  Port=4
  CURRENT_GEAR : Inport  Port=5
  FrntWiprSwtSts : Inport  Port=6
  WiprReq : Inport  Port=7
  FFogLmpSts_F_Pbox : Inport  Port=8
  LTurnLmpSwtSts : Inport  Port=9
  RTurnLmpSwtSts : Inport  Port=10
  VehYawRate : Inport  Port=11
  VehLatAccel : Inport  Port=12
  ABSActv : Inport  Port=13
  VDCActv : Inport  Port=14
  BTCActv : Inport  Port=15
  PTCActv : Inport  Port=16
  MSRActv : Inport  Port=17
  RFogLmpSts__Pbox : Inport  Port=18
  Compare To Constant{,1..3} (4 alike) : simulink/Logic and Bit Operations/Compare To Constant  relop=~=  const=1  OutDataTypeStr=boolean
  Constant1 : Constant  Value=P_AHBC_FOG_ENABLE
  Constant10 : Constant  Value=P_AHBC_WIPER_ENABLE
  Constant11 : Constant  Value=P_AHBC_FOG_ENABLE
  Constant13 : Constant  Value=P_AHBC_DRIVE_DIRECTION_ENABLE
  Constant2 : Constant  Value=P_AHBC_FOG_TIME
  Constant4 : Constant  Value=P_AHBC_WIPER_TIME
  Constant5 : Constant  Value=P_AHBC_FOG_TIME
  Constant7 : Constant  Value=P_AHBC_ESP_ENABLE
  Constant8 : Constant  Value=P_AHBC_ABS_ENABLE
  Constant9 : Constant  Value=P_AHBC_TURN_LAMP_ENABLE
  FodSSclc : Stateflow chart  TreatAsAtomicUnit=on
  FodSSclc1 : Stateflow chart  TreatAsAtomicUnit=on
  Logical Operator : Logic  Operator=OR  Inputs=4  AllPortsSameDT=off  OutDataTypeStr=boolean
  Logical Operator{1,7..12} (7 alike) : Logic  AllPortsSameDT=off  OutDataTypeStr=boolean
  Logical Operator2 : Logic  Operator=OR  Inputs=4  AllPortsSameDT=off  OutDataTypeStr=boolean
  Logical Operator3 : Logic  Operator=OR  AllPortsSameDT=off  OutDataTypeStr=boolean
  Logical Operator4 : Logic  Operator=OR  Inputs=3  AllPortsSameDT=off  OutDataTypeStr=boolean
  Logical Operator5 : Logic  Operator=OR  Inputs=4  AllPortsSameDT=off  OutDataTypeStr=boolean
  Logical Operator6 : Logic  Operator=OR  AllPortsSameDT=off  OutDataTypeStr=boolean
  Relay : Relay  OnSwitchValue=P_AHBC_YAW_RATE_ENTER  OffSwitchValue=P_AHBC_YAW_RATE_EXIT  OnOutputValue=true  OffOutputValue=false  OutDataTypeStr=boolean
  Relay1 : Relay  OnSwitchValue=P_AHBC_LAT_ACC_ENTER  OffSwitchValue=P_AHBC_LAT_ACC_EXIT  OnOutputValue=true  OffOutputValue=false  OutDataTypeStr=boolean
  Terminator : Terminator
  WiprSSclc : Stateflow chart  TreatAsAtomicUnit=on
  HighBeamSuppression : Outport
  LowPriorityTransformSuppression : Outport  Port=2
  HighPriorityTransformSuppression : Outport  Port=3
  wires:
  Constant2/1 -> FodSSclc1/2(HMA_FOG_TIME)
  Constant1/1 -> Logical Operator12/1
  Logical Operator12/1 -> Logical Operator/4  "RFogLmpSts"
  FodSSclc1/1(FogSS) -> Logical Operator12/2  "FogLmpSts_NC"
  RFogLmpSts__Pbox/1 -> FodSSclc1/1(RFogLmpSts__Pbox)
  CURRENT_GEAR/1 -> Terminator/1
  Logical Operator4/1 -> LowPriorityTransformSuppression/1  "AHBC_LowPriorityTransformSuppression"
  BTCActv/1 -> Logical Operator5/2
  PTCActv/1 -> Logical Operator5/3
  VehYawRate/1 -> Relay/1
  Logical Operator/1 -> HighBeamSuppression/1  "AHBC_HighBeamSuppression"
  FrntWiprSwtSts/1 -> WiprSSclc/1(FrntWiprSwtSts)
  FFogLmpSts_F_Pbox/1 -> FodSSclc/1(FFogLmpSts_F_Pbox)
  FLWheelDriveDirection/1 -> Compare To Constant/1
  WiprReq/1 -> WiprSSclc/2(WiprReq)
  Compare To Constant2/1 -> Logical Operator2/3
  ABSActv/1 -> Logical Operator11/2  "ABSSts_NC"
  RTurnLmpSwtSts/1 -> Logical Operator3/2
  Logical Operator11/1 -> Logical Operator6/1  "ABSSts"
  WiprSSclc/1(WiprSS) -> Logical Operator8/2  "WiprSts_NC"
  Compare To Constant3/1 -> Logical Operator2/4
  Logical Operator10/1 -> Logical Operator6/2  "ESPSts"
  Logical Operator2/1 -> Logical Operator1/2  "VehDirSsts_NC"
  FRWheelDriveDirection/1 -> Compare To Constant1/1
  LTurnLmpSwtSts/1 -> Logical Operator3/1
  FodSSclc/1(FogSS) -> Logical Operator7/2  "FogLmpSts_NC"
  MSRActv/1 -> Logical Operator5/4
  Relay1/1 -> Logical Operator4/3  "LatAccelSts"
  Logical Operator6/1 -> HighPriorityTransformSuppression/1  "AHBC_HighPriorityTransformSuppression"
  Compare To Constant1/1 -> Logical Operator2/2
  Constant8/1 -> Logical Operator11/1
  Logical Operator8/1 -> Logical Operator/2  "WiprSts"
  Constant7/1 -> Logical Operator10/1
  RLWheelDriveDirection/1 -> Compare To Constant2/1
  Logical Operator5/1 -> Logical Operator10/2  "ESPSts_NC"
  RRWheelDriveDirection/1 -> Compare To Constant3/1
  Logical Operator7/1 -> Logical Operator/3  "FFogLmpSts"
  Compare To Constant/1 -> Logical Operator2/1
  Relay/1 -> Logical Operator4/2  "YawRateSts"
  VehLatAccel/1 -> Relay1/1
  Logical Operator3/1 -> Logical Operator9/2  "TurnLmpSts_NC"
  Constant4/1 -> WiprSSclc/3(HMA_WIPER_TIME)
  Logical Operator1/1 -> Logical Operator/1  "VehDirSsts"
  Constant13/1 -> Logical Operator1/1
  Logical Operator9/1 -> Logical Operator4/1  "TurnLmpSts"
  VDCActv/1 -> Logical Operator5/1
  Constant9/1 -> Logical Operator9/1
  Constant11/1 -> Logical Operator7/1
  Constant10/1 -> Logical Operator8/1
  Constant5/1 -> FodSSclc/2(HMA_FOG_TIME)

== matlab function PvtSubSys_AHBC/Subsystem1/AHBC/ADB_adapter/MATLAB Function2 ==
  data: Target1_valid output boolean; Target2_valid output boolean; Target3_valid output boolean; Target4_valid output boolean; Target5_valid output boolean; Target6_valid output boolean
% function y = fcn(u)
% 
% y = u;
function [Target1_valid,Target2_valid,Target3_valid,Target4_valid,Target5_valid,Target6_valid]...
    =  XY()%Spots1HozlPosnLeAng,Spots1HozlPosnRiAng,Spots1Distance,  Spots2HozlPosnLeAng,  Spots2HozlPosnRiAng, ...
    %Spots2Distance,  Spots3HozlPosnLeAng,  Spots3HozlPosnRiAng,  Spots3Distance,  Spots4HozlPosnLeAng, ...
%Spots4HozlPosnRiAng,  Spots4Distance,  Spots5HozlPosnLeAng,  Spots5HozlPosnRiAng,  Spots5Distance,  ...
%Spots6HozlPosnLeAng,  Spots6HozlPosnRiAng,  Spots6Distance

  Target1_valid = true;
  Target2_valid = true;
  Target3_valid = true;
  Target4_valid = true;
  Target5_valid = true;
  Target6_valid = true;
  
%   LSVx1l=sin(Spots1HozlPosnLeAng/57.3)*single(Spots1Distance);
%   LSVx2l=sin( Spots2HozlPosnLeAng/57.3)* single(Spots2Distance) ;
%   LSVx3l=sin(Spots3HozlPosnLeAng/57.3 )* single(Spots3Distance );
%   LSVx4l=sin( Spots4HozlPosnLeAng/57.3)* single(Spots4Distance);
%   LSVx5l=sin(Spots5HozlPosnLeAng/57.3 )* single(Spots5Distance) ;
%   LSVx6l=sin( Spots6HozlPosnLeAng/57.3 )* single(Spots6Distance) ;
%   LSVx1r=sin( Spots1HozlPosnRiAng /57.3)* single(Spots1Distance) ;
%   LSVx2r=sin(Spots2HozlPosnRiAng/57.3)* single(Spots2Distance );
%   LSVx3r=sin( Spots3HozlPosnRiAng /57.3)* single(Spots3Distance) ;
%   LSVx4r=sin( Spots4HozlPosnRiAng /57.3)* single(Spots4Distance);
%   LSVx5r=sin( Spots5HozlPosnRiAng /57.3)* single(Spots5Distance) ;
%   LSVx6r=sin( Spots6HozlPosnRiAng /57.3)* single(Spots6Distance );
%   
%   if (LSVx1r-LSVx1l)>0.3 && (LSVx1r-LSVx1l)<6.5
%       Target1_valid = true;
%   end
%   if (LSVx2r-LSVx2l)>0.3 && (LSVx2r-LSVx2l)<6.5
%       Target2_valid = true;
%   end
%   if (LSVx3r-LSVx3l)>0.3 && (LSVx3r-LSVx3l)<6.5
%       Target3_valid = true;
%   end
%   if (LSVx4r-LSVx4l)>0.3 && (LSVx4r-LSVx4l)<6.5
%       Target4_valid = true;
%   end
%   if (LSVx5r-LSVx5l)>0.3 && (LSVx5r-LSVx5l)<6.5
%       Target5_valid = true;
%   end
%   if (LSVx6r-LSVx6l)>0.3 && (LSVx6r-LSVx6l)<6.5
%       Target6_valid = true;
%   end

end

== stateflow chart PvtSubSys_AHBC/Subsystem1/AHBC/ADB/Subsystem1/ADB_SM ==
  state ADB_OFF
    CamerSts=0;
  state ADB_ON
    state NotAvailableForADB
      du:CamerSts=0;
    state AvailableForADB
      du:CamerSts=1
    (default) -> NotAvailableForADB
    NotAvailableForADB -> AvailableForADB : [LSV_Running_Mode==3]
    AvailableForADB -> NotAvailableForADB : [(LSV_Running_Mode==1)...
        | ||(LSV_Running_Mode==2)]
  state Fault
    du:CamerSts=2;
  (default) -> ADB_OFF
  ADB_OFF -> ADB_ON : [VehConfigADB]
  ADB_ON -> ADB_OFF [order 1] : [~VehConfigADB]
  ADB_ON -> Fault [order 2] : [ADB_Error==1]
  Fault -> ADB_ON : [ADB_Error==0]
  data: LSV_Running_Mode input uint8; ADB_Error input uint8; VehConfigADB input uint8; CamerSts output uint8; i local uint8

== matlab function PvtSubSys_AHBC/Subsystem1/AHBC/ADB_adapter/MATLAB Function ==
  data: LSV_Vehicles_Count input; LSV_valid_state1 output uint8; LSV_valid_state2 output uint8; LSV_valid_state3 output uint8; LSV_valid_state4 output uint8; LSV_valid_state5 output uint8; LSV_valid_state6 output uint8; LSR_Strong_Reflectors_Count input; LSR_valid_state1 output uint8; LSR_valid_state2 output uint8; LSV_Distance1 input; LSV_Distance2 input; LSV_Distance3 input; LSV_Distance4 input; LSV_Distance5 input; LSV_Distance6 input; LSR_Distance1 input; LSR_Distance2 input; Target1_valid input boolean; Target2_valid input boolean; Target3_valid input boolean; Target4_valid input boolean; Target5_valid input boolean; Target6_valid input boolean
function [LSV_valid_state1,LSV_valid_state2,LSV_valid_state3,LSV_valid_state4,LSV_valid_state5,LSV_valid_state6,LSR_valid_state1,LSR_valid_state2]...
    = Elem_valid_Decide( LSV_Vehicles_Count,LSR_Strong_Reflectors_Count,LSV_Distance1,LSV_Distance2,LSV_Distance3,LSV_Distance4,LSV_Distance5,LSV_Distance6,LSR_Distance1,LSR_Distance2,...
    Target1_valid,Target2_valid,Target3_valid,Target4_valid,Target5_valid,Target6_valid)

LSV_valid_state1=uint8(0);
LSV_valid_state2=uint8(0);
LSV_valid_state3=uint8(0);
LSV_valid_state4=uint8(0);
LSV_valid_state5=uint8(0);
LSV_valid_state6=uint8(0);
LSR_valid_state1=uint8(0);
LSR_valid_state2=uint8(0);

% function [LSV_valid_state1,LSV_valid_state2,LSV_valid_state3,LSV_valid_state4,LSV_valid_state5,LSV_valid_state6]=LSV_Valid(LSV_Vehicles_Count)
if LSV_Vehicles_Count==0
    LSV_valid_state1=uint8(0);
    LSV_valid_state2=uint8(0);
    LSV_valid_state3=uint8(0);
    LSV_valid_state4=uint8(0);
    LSV_valid_state5=uint8(0);
    LSV_valid_state6=uint8(0);
else if LSV_Vehicles_Count==1 
        if LSV_Distance1<uint16(520) %%&& Target1_valid == true
            LSV_valid_state1=uint8(1);
        else
            LSV_valid_state1=uint8(0);
        end
    LSV_valid_state2=uint8(0);
    LSV_valid_state3=uint8(0);
    LSV_valid_state4=uint8(0);
    LSV_valid_state5=uint8(0);
    LSV_valid_state6=uint8(0);
else if LSV_Vehicles_Count==2
        if LSV_Distance1<uint16(520) %%&& Target1_valid == true
            LSV_valid_state1=uint8(1);
        else
            LSV_valid_state1=uint8(0);
        end
        if LSV_Distance2<uint16(520) %%&& Target2_valid == true
            LSV_valid_state2=uint8(1);
        else
            LSV_valid_state2=uint8(0);
        end
    LSV_valid_state3=uint8(0);
    LSV_valid_state4=uint8(0);
    LSV_valid_state5=uint8(0);
    LSV_valid_state6=uint8(0);
else if LSV_Vehicles_Count==3
       if LSV_Distance1<uint16(520) %%&& Target1_valid == true
            LSV_valid_state1=uint8(1);
        else
            LSV_valid_state1=uint8(0);
       end 
        if LSV_Distance2<uint16(520) %%&& Target2_valid == true
            LSV_valid_state2=uint8(1);
        else
            LSV_valid_state2=uint8(0);
        end 
       if LSV_Distance3<uint16(520) %%&& Target3_valid == true
            LSV_valid_state3=uint8(1);
        else
            LSV_valid_state3=uint8(0);
       end 
    LSV_valid_state4=uint8(0);
    LSV_valid_state5=uint8(0);
    LSV_valid_state6=uint8(0);
else if LSV_Vehicles_Count==4
       if LSV_Distance1<uint16(520) %%&& Target1_valid == true
            LSV_valid_state1=uint8(1);
        else
            LSV_valid_state1=uint8(0);
       end 
        if LSV_Distance2<uint16(520) %%&& Target2_valid == true
            LSV_valid_state2=uint8(1);
        else
            LSV_valid_state2=uint8(0);
        end 
       if LSV_Distance3<uint16(520) %%&& Target3_valid == true
            LSV_valid_state3=uint8(1);
        else
            LSV_valid_state3=uint8(0);
       end 
       if LSV_Distance4<uint16(520) %%&& Target4_valid == true
            LSV_valid_state4=uint8(1);
        else
            LSV_valid_state4=uint8(0);
       end
    LSV_valid_state5=uint8(0);
    LSV_valid_state6=uint8(0);
else if LSV_Vehicles_Count==5
       if LSV_Distance1<uint16(520) %%&& Target1_valid == true
            LSV_valid_state1=uint8(1);
        else
            LSV_valid_state1=uint8(0);
       end 
        if LSV_Distance2<uint16(520) %%&& Target2_valid == true
            LSV_valid_state2=uint8(1);
        else
            LSV_valid_state2=uint8(0);
        end 
       if LSV_Distance3<uint16(520) %%&& Target3_valid == true
            LSV_valid_state3=uint8(1);
        else
            LSV_valid_state3=uint8(0);
       end 
       if LSV_Distance4<uint16(520) %%&& Target4_valid == true
            LSV_valid_state4=uint8(1);
        else
            LSV_valid_state4=uint8(0);
       end
       if LSV_Distance5<uint16(520) %%&& Target5_valid == true
            LSV_valid_state5=uint8(1);
        else
            LSV_valid_state5=uint8(0);
       end
    LSV_valid_state6=uint8(0);
else if LSV_Vehicles_Count==6
       if LSV_Distance1<uint16(520) %%&& Target1_valid == true
            LSV_valid_state1=uint8(1);
        else
            LSV_valid_state1=uint8(0);
       end 
        if LSV_Distance2<uint16(520) %%&& Target2_valid == true
            LSV_valid_state2=uint8(1);
        else
            LSV_valid_state2=uint8(0);
        end 
       if LSV_Distance3<uint16(520) %%&& Target3_valid == true
            LSV_valid_state3=uint8(1);
        else
            LSV_valid_state3=uint8(0);
       end 
       if LSV_Distance4<uint16(520) %%&& Target4_valid == true
            LSV_valid_state4=uint8(1);
        else
            LSV_valid_state4=uint8(0);
       end
       if LSV_Distance5<uint16(520) %%&& Target5_valid == true
            LSV_valid_state5=uint8(1);
        else
            LSV_valid_state5=uint8(0);
       end
       if LSV_Distance6<uint16(520) %%&& Target6_valid == true
            LSV_valid_state6=uint8(1);
        else
            LSV_valid_state6=uint8(0);
       end
    end
    end
    end
    end
    end
    end
end

% function [LSR_valid_state1,LSR_valid_state2]=LSR_Valid(LSR_Strong_Reflectors_Count)
if LSR_Strong_Reflectors_Count==0
        LSR_valid_state1=uint8(0);
        LSR_valid_state2=uint8(0);
    else if LSR_Strong_Reflectors_Count==1
            if LSR_Distance1<uint16(520)
                LSR_valid_state1=uint8(1);
            else
                LSR_valid_state1=uint8(0);
            end
        LSR_valid_state2=uint8(0);
    else if LSR_Strong_Reflectors_Count==2
            if LSR_Distance1<uint16(520)
                LSR_valid_state1=uint8(1);
            else
                LSR_valid_state1=uint8(0);
            end
            if LSR_Distance2<uint16(520)
                LSR_valid_state2=uint8(1);
            else
                LSR_valid_state2=uint8(0);
            end

        end
    end
    end
end
